simulink model "Throttle_Position_Sensor"  (R2024a)
settings: Solver=VariableStepAuto  StartTime=0.0  StopTime=3  RelTol=1e-3
libraries: SignalEditorBlockLib x1
settings Model: Creator=VICTUS  LastModifiedBy=VICTUS

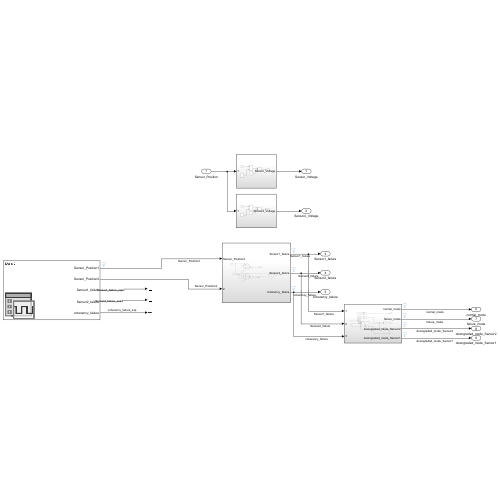
[thumbnail: Simulink's stored preview of the top-level diagram]
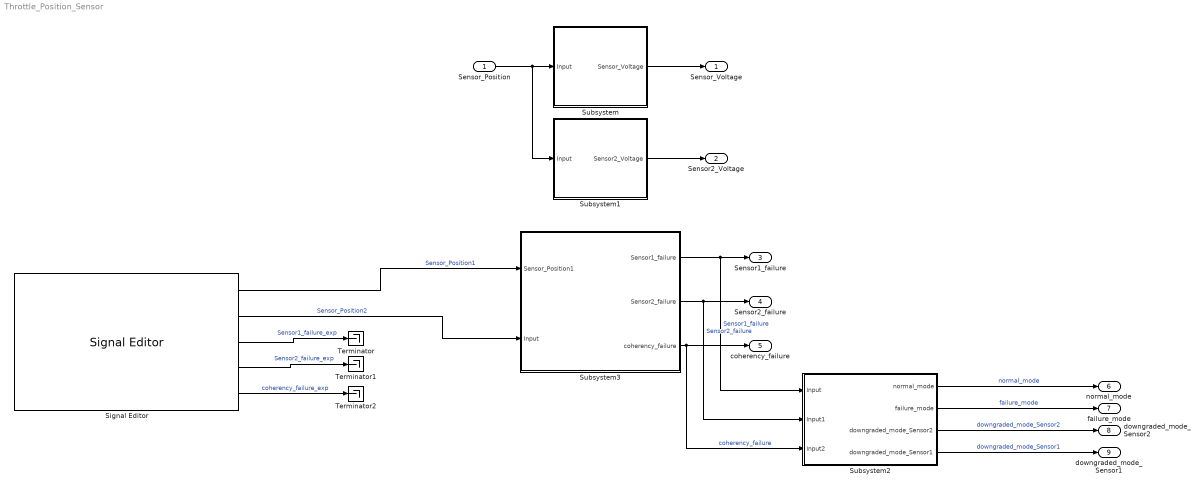
== system Throttle_Position_Sensor ==
  Sensor_Position : Inport
  Signal Editor : SignalEditorBlockLib/Signal Editor  FileName=Data.mat  ActiveScenario=Sheet2  ActiveSignal=Sensor_Position1  IsBus=off  OutputBusObjectStr=Bus: BusObject  SampleTime=0  Interpolate=off  ZeroCross=off  OutputAfterFinalValue=Setting to zero  Unit=inherit  PreserveSignalName=on  ApplySigPropsToAllScenarios=off  ApplySigPropsToAllSignals=off
  Subsystem : Subsystem
  Subsystem1 : Subsystem
  Subsystem2 : Subsystem
  Subsystem3 : Subsystem
  Terminator : Terminator
  Terminator1 : Terminator
  Terminator2 : Terminator
  Sensor_Voltage : Outport
  Sensor2_Voltage : Outport  Port=2
  Sensor1_failure : Outport  Port=3  OutDataTypeStr=boolean
  Sensor2_failure : Outport  Port=4  OutDataTypeStr=boolean
  coherency_failure : Outport  Port=5  OutDataTypeStr=boolean
  normal_mode : Outport  Port=6  OutDataTypeStr=boolean
  failure_mode : Outport  Port=7  OutDataTypeStr=boolean
  downgraded_mode_Sensor2 : Outport  Port=8  OutDataTypeStr=boolean
  downgraded_mode_Sensor1 : Outport  Port=9  OutDataTypeStr=boolean
  wires:
  Sensor_Position/1 -> Subsystem1/1(Input), Subsystem/1(Input)
  Signal Editor/1 -> Subsystem3/1(Sensor_Position1)  "Sensor_Position1"
  Subsystem3/2(Sensor2_failure) -> Subsystem2/2(Input1), Sensor2_failure/1  "Sensor2_failure"
  Subsystem3/1(Sensor1_failure) -> Subsystem2/1(Input), Sensor1_failure/1  "Sensor1_failure"
  Subsystem3/3(coherency_failure) -> Subsystem2/3(Input2), coherency_failure/1  "coherency_failure"
  Subsystem/1(Sensor_Voltage) -> Sensor_Voltage/1
  Subsystem1/1(Sensor2_Voltage) -> Sensor2_Voltage/1
  Signal Editor/2 -> Subsystem3/2(Input)  "Sensor_Position2"
  Signal Editor/3 -> Terminator/1  "Sensor1_failure_exp"
  Signal Editor/4 -> Terminator1/1  "Sensor2_failure_exp"
  Signal Editor/5 -> Terminator2/1  "coherency_failure_exp"
  Subsystem2/2(failure_mode) -> failure_mode/1  "failure_mode"
  Subsystem2/1(normal_mode) -> normal_mode/1  "normal_mode"
  Subsystem2/3(downgraded_mode_Sensor2) -> downgraded_mode_Sensor2/1  "downgraded_mode_Sensor2"
  Subsystem2/4(downgraded_mode_Sensor1) -> downgraded_mode_Sensor1/1  "downgraded_mode_Sensor1"

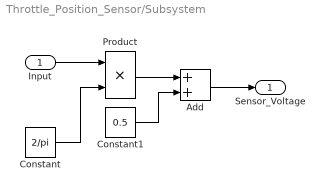
== system Throttle_Position_Sensor/Subsystem ==
  Input : Inport
  Add : Sum
  Constant : Constant  Value=2/pi
  Constant1 : Constant  Value=0.5
  Product : Product
  Sensor_Voltage : Outport
  wires:
  Input/1 -> Product/1
  Constant/1 -> Product/2
  Product/1 -> Add/1
  Add/1 -> Sensor_Voltage/1
  Constant1/1 -> Add/2

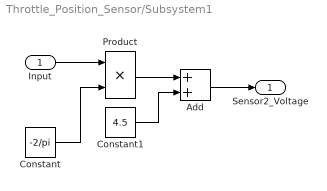
== system Throttle_Position_Sensor/Subsystem1 ==
  Input : Inport
  Add : Sum
  Constant : Constant  Value=-2/pi
  Constant1 : Constant  Value=4.5
  Product : Product
  Sensor2_Voltage : Outport
  wires:
  Constant1/1 -> Add/2
  Add/1 -> Sensor2_Voltage/1
  Product/1 -> Add/1
  Constant/1 -> Product/2
  Input/1 -> Product/1

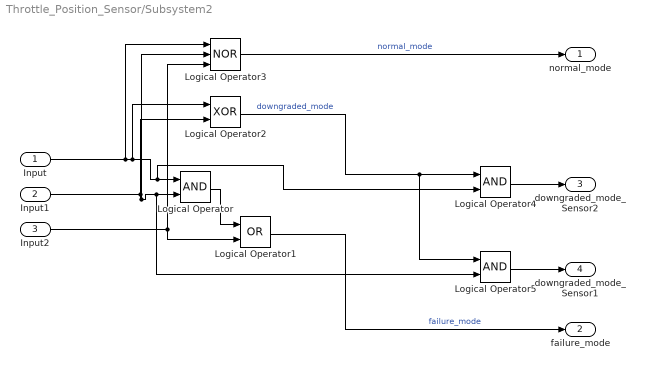
== system Throttle_Position_Sensor/Subsystem2 ==
  Input : Inport
  Input1 : Inport  Port=2
  Input2 : Inport  Port=3
  Logical Operator : Logic  AllPortsSameDT=off  OutDataTypeStr=boolean
  Logical Operator1 : Logic  Operator=OR  AllPortsSameDT=off  OutDataTypeStr=boolean
  Logical Operator2 : Logic  Operator=XOR  AllPortsSameDT=off  OutDataTypeStr=boolean
  Logical Operator3 : Logic  Operator=NOR  Inputs=3  AllPortsSameDT=off  OutDataTypeStr=boolean
  Logical Operator4 : Logic  AllPortsSameDT=off  OutDataTypeStr=boolean
  Logical Operator5 : Logic  AllPortsSameDT=off  OutDataTypeStr=boolean
  normal_mode : Outport
  failure_mode : Outport  Port=2  OutDataTypeStr=boolean
  downgraded_mode_Sensor2 : Outport  Port=3
  downgraded_mode_Sensor1 : Outport  Port=4
  wires:
  Input/1 -> Logical Operator3/1, Logical Operator2/1, Logical Operator4/2, Logical Operator/1
  Input1/1 -> Logical Operator3/2, Logical Operator5/2, Logical Operator/2, Logical Operator2/2
  Logical Operator/1 -> Logical Operator1/1
  Input2/1 -> Logical Operator1/2, Logical Operator3/3
  Logical Operator1/1 -> failure_mode/1  "failure_mode"
  Logical Operator2/1 -> Logical Operator5/1, Logical Operator4/1  "downgraded_mode"
  Logical Operator3/1 -> normal_mode/1  "normal_mode"
  Logical Operator4/1 -> downgraded_mode_Sensor2/1
  Logical Operator5/1 -> downgraded_mode_Sensor1/1

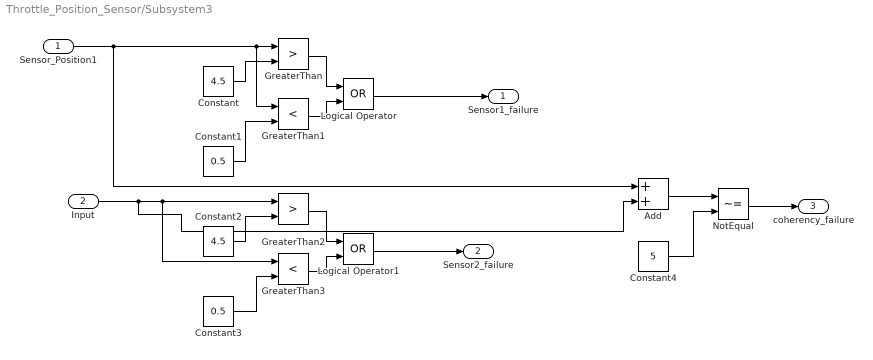
== system Throttle_Position_Sensor/Subsystem3 ==
  Sensor_Position1 : Inport  OutDataTypeStr=double
  Input : Inport  Port=2  OutDataTypeStr=double
  Add : Sum
  Constant : Constant  Value=4.5
  Constant1 : Constant  Value=0.5
  Constant2 : Constant  Value=4.5
  Constant3 : Constant  Value=0.5
  Constant4 : Constant  Value=5
  GreaterThan : RelationalOperator  Operator=>  OutDataTypeStr=boolean  RndMeth=Simplest  InputSameDT=off
  GreaterThan1 : RelationalOperator  Operator=<  OutDataTypeStr=boolean  RndMeth=Simplest  InputSameDT=off
  GreaterThan2 : RelationalOperator  Operator=>  OutDataTypeStr=boolean  RndMeth=Simplest  InputSameDT=off
  GreaterThan3 : RelationalOperator  Operator=<  OutDataTypeStr=boolean  RndMeth=Simplest  InputSameDT=off
  Logical Operator : Logic  Operator=OR  AllPortsSameDT=off  OutDataTypeStr=boolean
  Logical Operator1 : Logic  Operator=OR  AllPortsSameDT=off  OutDataTypeStr=boolean
  NotEqual : RelationalOperator  Operator=~=  OutDataTypeStr=boolean  RndMeth=Simplest  InputSameDT=off
  Sensor1_failure : Outport
  Sensor2_failure : Outport  Port=2
  coherency_failure : Outport  Port=3
  wires:
  GreaterThan/1 -> Logical Operator/1
  GreaterThan1/1 -> Logical Operator/2
  Constant/1 -> GreaterThan/2
  Logical Operator/1 -> Sensor1_failure/1
  Constant1/1 -> GreaterThan1/2
  Logical Operator1/1 -> Sensor2_failure/1
  Constant2/1 -> GreaterThan2/2
  Sensor_Position1/1 -> Add/1, GreaterThan1/1, GreaterThan/1
  Constant3/1 -> GreaterThan3/2
  GreaterThan3/1 -> Logical Operator1/2
  GreaterThan2/1 -> Logical Operator1/1
  Add/1 -> NotEqual/1
  Constant4/1 -> NotEqual/2
  NotEqual/1 -> coherency_failure/1
  Input/1 -> Add/2, GreaterThan3/1, GreaterThan2/1
